simulink model "tqdtqr_rebuild_V3"  (R2021b)
settings: Solver=VariableStepAuto  StartTime=0.0  StopTime=10.0  RelTol=1e-3
undefined symbols (not defined in the file): ATQD_AfterTqMinGain_X_Deg, ATQD_APSCreepBaseTqD_X_kph, ATQD_APSCreepBaseTqD_Y_Deg, ATQD_APSCreepBaseTqR_X_kph, ATQD_APSCreepBaseTqR_Y_Deg, ATQD_APSCreepIterm_X_kph, ATQD_APSCreepIterm_Y_kph, ATQD_APSCreepPterm_X_kph, ATQD_APSCreepPterm_Y_kph, ATQD_APSDecReq_X_kph, ATQD_APSDecReq_Y_mps2, ATQD_APSDecReqCMD_X_kph, ATQD_APSDecReqTs_X_pct, ATQD_APSDecTimeGain_X_Deg, ATQD_APSDecTimeGain_Y_s, ATQD_APSReqLowSpd_X_Deg, ATQD_AutoHoldReleaseBPS_X_Deg, ATQD_AWDLoadTrqnsGain_X_kg, ATQD_AWDLoadTrqnsGain_Y_pct, ATQD_BOSEnBPSPosn_X_kph, ATQD_BOSMap_X_rpm, ATQD_BOSMap_Y_pct, ATQD_CreepBaseTqD_X_kph, ATQD_CreepBaseTqD_Y_Deg, ATQD_CreepBaseTqR_X_kph, ATQD_CreepBaseTqR_Y_Deg, ATQD_CreepBPSDisPosn_X_Deg, ATQD_CreepBPSDisPosnR_X_Deg, ATQD_CreepBPSEnPosn_X_Deg, ATQD_CreepBPSEnPosnR_X_Deg, ATQD_CreepDeltaTq_X_kph, ATQD_CreepIterm_X_kph, ATQD_CreepIterm_Y_kph, ATQD_CreepItermMaxLimit_X_pct, ATQD_CreepPreloadTime_X_kph, ATQD_CreepPreloadTq_X_kph, ATQD_CreepPreloadTq_Y_s, ATQD_CreepProtTq_X_Deg, ATQD_CreepPterm_X_kph, ATQD_CreepPterm_Y_kph, ATQD_CreepRrTqSpRat_X_rpm, ATQD_CreepRrTqSpRat_Y_Nm, ATQD_CreepTargetSpdD_X_pct, ATQD_CreepTargetSpdR_X_pct, ATQD_CreepUpLimitTq_X_rpm, ATQD_DecIneOPDHoldEnDelay_X_Deg, ATQD_DecIneOPDHoldEnDelay_Y_bar, ATQD_ECOTqMapD_X_rpm, ATQD_ECOTqMapD_Y_pct, ATQD_EMTqMapD_X_rpm, ATQD_EMTqMapD_Y_pct, ATQD_EOPDTqMapDCon_X_rpm, ATQD_EOPDTqMapDCon_Y_Deg, ATQD_EstInitVehWeight_X_c, ATQD_FAfterTqCMDGain_X_rpm, ATQD_FAfterTqCMDGain_Y_pct, ATQD_ForceLowSpd_X_Deg, ATQD_ForcePLimitSpd_X_Deg, ATQD_FrLossMAPLowV_X_rpm, ATQD_FrLossMAPLowV_Y_Nm ... (+949)
libraries: simulink x235, hcu_lib x208, tqr x63, tqd x6
(part 4 of 37)

== system tqdtqr_rebuild_V3/Input_Convert/Main function ==
  note: --------------------------------------------------------------------TQR----------------------------------------------------------------
  BSCPIn_outputs : Inport
  BSignalConvert_outputs : Inport  Port=2
  BFunction_outputs : Inport  Port=3
  BMain_outputs : Inport  Port=4
  Add B regen to ramp enable judge : Subsystem
  AvaliableTqLimit function : Subsystem
  Bus Creator : BusCreator  Inputs=72
  DriverWhlTqDem function : Subsystem
  Front/Rear EDU Tq Up/Low Limit : Subsystem
  Front/Rear ramp parameters determine : Subsystem
  Front/Rear wheel torque different function : Subsystem
  Front/Rear wheel torque limitation determine function : Subsystem
  Front/Rear zero point transfer : Subsystem
  Gear detection to inverse motor : Subsystem
  Tq coordination function : Subsystem
  Tq distribution function : Subsystem
  MainFunction_outputs : Outport
  wires:
  [BSCPIn_outputs] -> Tq distribution function/1(BSCPIn_outputs)
  [BSignalConvert_outputs] -> DriverWhlTqDem function/2(BSignalConvert_outputs)
  [BMain_outputs] -> Tq distribution function/2(BMain_outputs)
  [BFunction_outputs] -> Tq distribution function/4(BFunction_outputs)
  [BSignalConvert_outputs] -> Tq distribution function/3(BSignalConvert_outputs)
  [BSCPIn_outputs] -> Tq coordination function/1(BSCPIn_outputs)
  [BSignalConvert_outputs] -> Tq coordination function/2(BSignalConvert_outputs)
  [BFunction_outputs] -> DriverWhlTqDem function/3(BFunction_outputs)
  [BSCPIn_outputs] -> DriverWhlTqDem function/1(BSCPIn_outputs)
  BSCPIn_outputs/1 -> [BSCPIn_outputs]
  BFunction_outputs/1 -> [BFunction_outputs]
  BSignalConvert_outputs/1 -> [BSignalConvert_outputs]
  BMain_outputs/1 -> [BMain_outputs]
  [BMain_outputs] -> Tq coordination function/3(BMain_outputs)
  [BSCPIn_outputs] -> AvaliableTqLimit function/1(BSCPIn_outputs)
  [BSignalConvert_outputs] -> AvaliableTqLimit function/2(BSignalConvert_outputs)
  [BFunction_outputs] -> AvaliableTqLimit function/3(BFunction_outputs)
  [BMain_outputs] -> AvaliableTqLimit function/4(BMain_outputs)
  [BMain_outputs] -> DriverWhlTqDem function/4(BMain_outputs)
  DriverWhlTqDem function/1(VTQD_RollRegenEnable_flg) -> [VTQD_RollRegenEnable_flg]
  DriverWhlTqDem function/2(VTQD_BOSEnable_flg) -> [VTQD_BOSEnable_flg]
  DriverWhlTqDem function/3(VTQD_BOSTq_Nm) -> [VTQD_BOSTq_Nm]
  DriverWhlTqDem function/4(VTQD_IVIRockModeEn_flg) -> [VTQD_IVIRockModeEn_flg]
  DriverWhlTqDem function/5(VTQD_LoSpdBrkCtrl_flg) -> [VTQD_LoSpdBrkCtrl_flg]
  DriverWhlTqDem function/6(VTQD_RockModeTCSReq_flg) -> [VTQD_RockModeTCSReq_flg]
  DriverWhlTqDem function/7(VTQD_RockModePedTq_Nm) -> [VTQD_RockModePedTq_Nm]
  DriverWhlTqDem function/8(VTQD_RockModeTqLim_flg) -> [VTQD_RockModeTqLim_flg]
  DriverWhlTqDem function/9(VTQD_PreLoadPreEn_flg) -> [VTQD_PreLoadPreEn_flg]
  DriverWhlTqDem function/10(VTQD_PreloadTq_Nm) -> [VTQD_PreloadTq_Nm]
  DriverWhlTqDem function/11(VTQD_PreLoadHold_flg) -> [VTQD_PreLoadHold_flg]
  DriverWhlTqDem function/12(VTQD_CreepWhlTqDem_Nm) -> [VTQD_CreepWhlTqDem_Nm]
  DriverWhlTqDem function/13(VTQD_CreepPrLoadEnable_flg) -> [VTQD_CreepPrLoadEnable_flg]
  DriverWhlTqDem function/14(VTQD_CreepProtTqEn_flg) -> [VTQD_CreepProtTqEn_flg]
  DriverWhlTqDem function/15(VTQD_PedalMapWhlTq_Nm) -> [VTQD_PedalMapWhlTq_Nm]
  DriverWhlTqDem function/16(VTQD_EVDriveModeValid_flg) -> [VTQD_EVDriveModeValid_flg]
  DriverWhlTqDem function/17(VTQD_RegenTqLimitEn_flg) -> [VTQD_RegenTqLimitEn_flg]
  DriverWhlTqDem function/18(VTQD_PedAccTqEn_flg) -> [VTQD_PedAccTqEn_flg]
  DriverWhlTqDem function/19(VTQD_SlideRegenLimTq_Nm) -> [VTQD_SlideRegenLimTq_Nm]
  DriverWhlTqDem function/20(VTQD_OPDOn2Off_flg) -> [VTQD_OPDOn2Off_flg]
  DriverWhlTqDem function/21(VTQD_CreepTCSActive_flg) -> [VTQD_CreepTCSActive_flg]
  DriverWhlTqDem function/22(VTQD_FrPreloadTq_Nm) -> [VTQD_FrPreloadTq_Nm]
  DriverWhlTqDem function/23(VTQD_RrPreloadTq_Nm) -> [VTQD_RrPreloadTq_Nm]
  DriverWhlTqDem function/24(VTQD_CreepEnable_flg) -> [VTQD_CreepEnable_flg]
  DriverWhlTqDem function/25(VTQD_CreepBaseTqD_Nm) -> [VTQD_CreepBaseTqD_Nm]
  [VTQD_RollRegenEnable_flg] -> Tq coordination function/4(VTQD_RollRegenEnable_flg)
  [VTQD_CreepPrLoadEnable_flg] -> Tq distribution function/5(VTQD_CreepPrLoadEnable_flg)
  [VTQD_CreepEnable_flg] -> Tq distribution function/6(VTQD_CreepEnable_flg)
  [VTQD_RrPreloadTq_Nm] -> Tq distribution function/7(VTQD_RrPreloadTq_Nm)
  [VTQD_FrPreloadTq_Nm] -> Tq distribution function/8(VTQD_FrPreloadTq_Nm)
  [VTQD_PreLoadHold_flg] -> Tq distribution function/9(VTQD_PreLoadHold_flg)
  Tq coordination function/1(VTQD_TqSourceFr_enum) -> [VTQD_TqSourceFr_enum]
  Tq coordination function/2(VTQD_TqSourceRr_enum) -> [VTQD_TqSourceRr_enum]
  Tq coordination function/3(VTQD_TotalWhlTqCapMot_Nm) -> [VTQD_TotalWhlTqCapMot_Nm]
  Tq coordination function/4(VTQD_TotalWhlTqCapGen_Nm) -> [VTQD_TotalWhlTqCapGen_Nm]
  [VTQD_TqSourceRr_enum] -> DriverWhlTqDem function/6(VTQD_TqSourceRr_enum)
  [VTQD_TqSourceFr_enum] -> DriverWhlTqDem function/5(VTQD_TqSourceFr_enum)
  Tq distribution function/1(VTQD_FrEDUSpRat_rat) -> [VTQD_FrEDUSpRat_rat]
  Tq distribution function/2(VTQD_RrEDUSpRat_rat) -> [VTQD_RrEDUSpRat_rat]
  Tq distribution function/3(VTQD_RockModePedTqFr_Nm) -> [VTQD_RockModePedTqFr_Nm]
  Tq distribution function/4(VTQD_RockModePedTqRr_Nm) -> [VTQD_RockModePedTqRr_Nm]
  Tq distribution function/5(VTQD_TMEnOutpTqSta_enum) -> [VTQD_TMEnOutpTqSta_enum]
  Tq distribution function/6(VTQD_NewDistFrWhlTq_Nm) -> [VTQD_NewDistFrWhlTq_Nm]
  Tq distribution function/7(VTQD_NewDistRrWhlTq_Nm) -> [VTQD_NewDistRrWhlTq_Nm]
  [VTQD_FrEDUSpRat_rat] -> AvaliableTqLimit function/6(VTQD_FrEDUSpRat_rat)
  [VTQD_RrEDUSpRat_rat] -> AvaliableTqLimit function/7(VTQD_RrEDUSpRat_rat)
  AvaliableTqLimit function/1(VTQD_WhlTqCapMotFr_Nm) -> [VTQD_WhlTqCapMotFr_Nm]
  AvaliableTqLimit function/2(VTQD_WhlTqCapMotRr_Nm) -> [VTQD_WhlTqCapMotRr_Nm]
  AvaliableTqLimit function/3(VTQD_WhlTqCapGenFr_Nm) -> [VTQD_WhlTqCapGenFr_Nm]
  AvaliableTqLimit function/4(VTQD_WhlTqCapGenRr_Nm) -> [VTQD_WhlTqCapGenRr_Nm]
  AvaliableTqLimit function/5(VTQD_MotorLossTotal_kw) -> [VTQD_MotorLossTotal_kw]
  AvaliableTqLimit function/6(VTQD_FAfterTqCMDGain_c) -> [VTQD_FAfterTqCMDGain_c]
  AvaliableTqLimit function/7(VTQD_RAfterTqCMDGain_c) -> [VTQD_RAfterTqCMDGain_c]
  [VTQD_MotorLossTotal_kw] -> Tq coordination function/5(VTQD_MotorLossTotal_kw)
  [VTQD_RollRegenEnable_flg] -> Bus Creator/1
  [VTQD_BOSEnable_flg] -> Bus Creator/2
  [VTQD_BOSTq_Nm] -> Bus Creator/3
  [VTQD_IVIRockModeEn_flg] -> Bus Creator/4
  [VTQD_LoSpdBrkCtrl_flg] -> Bus Creator/5
  [VTQD_RockModeTCSReq_flg] -> Bus Creator/6
  [VTQD_RockModePedTq_Nm] -> Bus Creator/7
  [VTQD_RockModeTqLim_flg] -> Bus Creator/8
  [VTQD_PreLoadPreEn_flg] -> Bus Creator/9
  [VTQD_PreloadTq_Nm] -> Bus Creator/10
  [VTQD_PreLoadHold_flg] -> Bus Creator/11
  [VTQD_CreepWhlTqDem_Nm] -> Bus Creator/12
  [VTQD_CreepPrLoadEnable_flg] -> Bus Creator/13
  [VTQD_CreepProtTqEn_flg] -> Bus Creator/14
  [VTQD_PedalMapWhlTq_Nm] -> Bus Creator/15
  [VTQD_EVDriveModeValid_flg] -> Bus Creator/16
  [VTQD_RegenTqLimitEn_flg] -> Bus Creator/17
  [VTQD_PedAccTqEn_flg] -> Bus Creator/18
  [VTQD_SlideRegenLimTq_Nm] -> Bus Creator/19
  [VTQD_OPDOn2Off_flg] -> Bus Creator/20
  [VTQD_CreepTCSActive_flg] -> Bus Creator/21
  [VTQD_FrPreloadTq_Nm] -> Bus Creator/22
  [VTQD_RrPreloadTq_Nm] -> Bus Creator/23
  [VTQD_CreepEnable_flg] -> Bus Creator/24
  [VTQD_CreepBaseTqD_Nm] -> Bus Creator/25
  [VTQD_TqSourceFr_enum] -> Bus Creator/26
  [VTQD_TqSourceRr_enum] -> Bus Creator/27
  [VTQD_TotalWhlTqCapMot_Nm] -> Bus Creator/28
  [VTQD_FrEDUSpRat_rat] -> Bus Creator/31
  [VTQD_RrEDUSpRat_rat] -> Bus Creator/32
  [VTQD_RockModePedTqFr_Nm] -> Bus Creator/33
  [VTQD_RockModePedTqRr_Nm] -> Bus Creator/34
  [VTQD_TMEnOutpTqSta_enum] -> Bus Creator/35
  [VTQD_NewDistFrWhlTq_Nm] -> Bus Creator/36
  [VTQD_NewDistRrWhlTq_Nm] -> Bus Creator/37
  [VTQD_WhlTqCapMotFr_Nm] -> Bus Creator/38
  [VTQD_WhlTqCapMotRr_Nm] -> Bus Creator/39
  [VTQD_WhlTqCapGenFr_Nm] -> Bus Creator/40
  [VTQD_WhlTqCapGenRr_Nm] -> Bus Creator/41
  [VTQD_MotorLossTotal_kw] -> Bus Creator/42
  [VTQD_FAfterTqCMDGain_c] -> Bus Creator/43
  [VTQD_RAfterTqCMDGain_c] -> Bus Creator/44
  Bus Creator/1 -> MainFunction_outputs/1
  [BSCPIn_outputs] -> Front/Rear wheel torque different function/1(BSCPIn_outputs)
  [BSignalConvert_outputs] -> Front/Rear wheel torque different function/2(BSignalConvert_outputs)
  Front/Rear wheel torque different function/1(VTQR_FShaftSpdTqLimCoe_c) -> [VTQR_FShaftSpdTqLimCoe_c]
  Front/Rear wheel torque different function/2(VTQR_FTimerTqLimCoe_c) -> [VTQR_FTimerTqLimCoe_c]
  Front/Rear wheel torque different function/3(VTQR_RShaftSpdTqLimCoe_c) -> [VTQR_RShaftSpdTqLimCoe_c]
  Front/Rear wheel torque different function/4(VTQR_RTimerTqLimCoe_c) -> [VTQR_RTimerTqLimCoe_c]
  [VTQR_FShaftSpdTqLimCoe_c] -> Front/Rear wheel torque limitation determine function/3(VTQR_FShaftSpdTqLimCoe_c)
  [VTQR_FTimerTqLimCoe_c] -> Front/Rear wheel torque limitation determine function/4(VTQR_FTimerTqLimCoe_c)
  [VTQR_RShaftSpdTqLimCoe_c] -> Front/Rear wheel torque limitation determine function/5(VTQR_RShaftSpdTqLimCoe_c)
  [VTQR_RTimerTqLimCoe_c] -> Front/Rear wheel torque limitation determine function/6(VTQR_RTimerTqLimCoe_c)
  [BMain_outputs] -> Front/Rear wheel torque limitation determine function/2(BMain_outputs)
  [BSCPIn_outputs] -> Front/Rear wheel torque limitation determine function/1(BSCPIn_outputs)
  Front/Rear wheel torque limitation determine function/1(VTQR_ActFEDUTrqUpLim_Nm) -> [VTQR_ActFEDUTrqUpLim_Nm]
  Front/Rear wheel torque limitation determine function/2(VTQR_ActFEDUTrqLowLim_Nm) -> [VTQR_ActFEDUTrqLowLim_Nm]
  Front/Rear wheel torque limitation determine function/4(VTQR_ActREDUTrqLowLim_Nm) -> [VTQR_ActREDUTrqLowLim_Nm]
  Front/Rear wheel torque limitation determine function/3(VTQR_ActREDUTrqUpLim_Nm) -> [VTQR_ActREDUTrqUpLim_Nm]
  Front/Rear wheel torque different function/5(VTQR_FShaftSpdTqLimLow_flg) -> [VTQR_FShaftSpdTqLimLow_flg]
  Front/Rear wheel torque different function/6(VTQR_FTimerTqLimLow_flg) -> [VTQR_FTimerTqLimLow_flg]
  Front/Rear wheel torque different function/7(VTQR_RShaftSpdTqLimLow_flg) -> [VTQR_RShaftSpdTqLimLow_flg]
  Front/Rear wheel torque different function/8(VTQR_RTimerTqLimLow_flg) -> [VTQR_RTimerTqLimLow_flg]
  [BSCPIn_outputs] -> Front/Rear zero point transfer/1(BSCPIn_outputs)
  [BMain_outputs] -> Front/Rear zero point transfer/3(BMain_outputs)
  [BSignalConvert_outputs] -> Front/Rear zero point transfer/2(BSignalConvert_outputs)
  [VTQD_CreepPrLoadEnable_flg] -> Front/Rear zero point transfer/4(VTQD_CreepPrLoadEnable_flg)
  [VTQD_PreLoadPreEn_flg] -> Front/Rear zero point transfer/5(VTQD_PreLoadPreEn_flg)
  Front/Rear zero point transfer/1(VTQR_FrTqZeroTransUpBound_Nm) -> [VTQR_FrTqZeroTransUpBound_Nm]
  Front/Rear zero point transfer/2(VTQR_FrTqZeroTransLowBound_Nm) -> [VTQR_FrTqZeroTransLowBound_Nm]
  Front/Rear zero point transfer/3(VTQR_FrTqZeroTrans_enum) -> [VTQR_FrTqZeroTrans_enum]
  Front/Rear zero point transfer/4(VTQR_RrTqZeroTransUpBound_Nm) -> [VTQR_RrTqZeroTransUpBound_Nm]
  Front/Rear zero point transfer/5(VTQR_RrTqZeroTransLowBound_Nm) -> [VTQR_RrTqZeroTransLowBound_Nm]
  Front/Rear zero point transfer/6(VTQR_RrTqZeroTrans_enum) -> [VTQR_RrTqZeroTrans_enum]
  [VTQR_FShaftSpdTqLimLow_flg] -> Bus Creator/45
  [VTQR_FTimerTqLimLow_flg] -> Bus Creator/46
  [VTQR_RShaftSpdTqLimLow_flg] -> Bus Creator/47
  [VTQR_RTimerTqLimLow_flg] -> Bus Creator/48
  [VTQR_ActFEDUTrqUpLim_Nm] -> Bus Creator/49
  [VTQR_ActFEDUTrqLowLim_Nm] -> Bus Creator/50
  [VTQR_ActREDUTrqUpLim_Nm] -> Bus Creator/51
  [VTQR_ActREDUTrqLowLim_Nm] -> Bus Creator/52
  [VTQR_FrTqZeroTransUpBound_Nm] -> Bus Creator/53
  [VTQR_FrTqZeroTransLowBound_Nm] -> Bus Creator/54
  [VTQR_FrTqZeroTrans_enum] -> Bus Creator/55
  [VTQR_RrTqZeroTransUpBound_Nm] -> Bus Creator/56
  [VTQR_RrTqZeroTransLowBound_Nm] -> Bus Creator/57
  [VTQR_RrTqZeroTrans_enum] -> Bus Creator/58
  [BFunction_outputs] -> Gear detection to inverse motor/1(BFunction_outputs)
  [BMain_outputs] -> Gear detection to inverse motor/2(BMain_outputs)
  Gear detection to inverse motor/1(VTQR_FrGearChange_flg) -> [VTQR_FrGearChange_flg]
  Gear detection to inverse motor/2(VTQR_RrGearChange_flg) -> [VTQR_RrGearChange_flg]
  [VTQR_FrGearChange_flg] -> Bus Creator/59
  [VTQR_RrGearChange_flg] -> Bus Creator/60
  [BSignalConvert_outputs] -> Front/Rear ramp parameters determine/2(BSignalConvert_outputs)
  [BSCPIn_outputs] -> Front/Rear ramp parameters determine/1(BSCPIn_outputs)
  [VTQD_RollRegenEnable_flg] -> Front/Rear ramp parameters determine/5(VTQD_RollRegenEnable_flg)
  [VTQD_TqSourceFr_enum] -> Front/Rear ramp parameters determine/6(VTQD_TqSourceFr_enum)
  [BMain_outputs] -> Front/Rear ramp parameters determine/4(BMain_outputs)
  [VTQD_EVDriveModeValid_flg] -> Front/Rear ramp parameters determine/7(VTQD_EVDriveModeValid_flg)
  [VTQD_PreLoadHold_flg] -> Front/Rear ramp parameters determine/8(VTQD_PreLoadHold_flg)
  [VTQD_CreepPrLoadEnable_flg] -> Front/Rear ramp parameters determine/9(VTQD_CreepPrLoadEnable_flg)
  [VTQD_PedAccTqEn_flg] -> Front/Rear ramp parameters determine/10(VTQD_PedAccTqEn_flg)
  [VTQD_PreLoadPreEn_flg] -> Front/Rear ramp parameters determine/11(VTQD_PreLoadPreEn_flg)
  [VTQD_IVIRockModeEn_flg] -> Front/Rear ramp parameters determine/12(VTQD_IVIRockModeEn_flg)
  [VTQR_FrTqZeroTrans_enum] -> Front/Rear ramp parameters determine/13(VTQR_FrTqZeroTrans_enum)
  [VTQD_RegenTqLimitEn_flg] -> Front/Rear ramp parameters determine/14(VTQD_RegenTqLimitEn_flg)
  [BFunction_outputs] -> Front/Rear ramp parameters determine/3(BFunction_outputs)
  [VTQD_TqSourceRr_enum] -> Front/Rear ramp parameters determine/15(VTQD_TqSourceRr_enum)
  [VTQR_RrTqZeroTrans_enum] -> Front/Rear ramp parameters determine/16(VTQR_RrTqZeroTrans_enum)
  Front/Rear ramp parameters determine/1(VTQR_FrFirstOrderInpTs_c) -> [VTQR_FrFirstOrderInpTs_c]
  Front/Rear ramp parameters determine/2(VTQR_FrRateLimitInc_Nm) -> [VTQR_FrRateLimitInc_Nm]
  Front/Rear ramp parameters determine/3(VTQR_FrRateLimitDec_Nm) -> [VTQR_FrRateLimitDec_Nm]
  Front/Rear ramp parameters determine/4(VTQR_RrFirstOrderInpTs_c) -> [VTQR_RrFirstOrderInpTs_c]
  Front/Rear ramp parameters determine/5(VTQR_RrRateLimitInc_Nm) -> [VTQR_RrRateLimitInc_Nm]
  Front/Rear ramp parameters determine/6(VTQR_RrRateLimitDec_Nm) -> [VTQR_RrRateLimitDec_Nm]
  [VTQR_FrFirstOrderInpTs_c] -> Bus Creator/61
  [VTQR_FrRateLimitInc_Nm] -> Bus Creator/62
  [VTQR_FrRateLimitDec_Nm] -> Bus Creator/63
  [VTQR_RrFirstOrderInpTs_c] -> Bus Creator/64
  [VTQR_RrRateLimitInc_Nm] -> Bus Creator/65
  [VTQR_RrRateLimitDec_Nm] -> Bus Creator/66
  [VTQR_FrTqZeroTransLowBound_Nm] -> Tq distribution function/10(VTQR_FrTqZeroTransLowBound_Nm)
  [VTQR_RrTqZeroTransLowBound_Nm] -> Tq distribution function/11(VTQR_RrTqZeroTransLowBound_Nm)
  [VTQR_FShaftSpdTqLimLow_flg] -> DriverWhlTqDem function/7(VTQR_FShaftSpdTqLimLow_flg)
  [VTQR_FTimerTqLimLow_flg] -> DriverWhlTqDem function/8(VTQR_FTimerTqLimLow_flg)
  [VTQR_RShaftSpdTqLimLow_flg] -> DriverWhlTqDem function/9(VTQR_RShaftSpdTqLimLow_flg)
  [VTQR_RTimerTqLimLow_flg] -> DriverWhlTqDem function/10(VTQR_RTimerTqLimLow_flg)
  [BSCPIn_outputs] -> Add B regen to ramp enable judge/1(BSCPIn_outputs)
  [BSignalConvert_outputs] -> Add B regen to ramp enable judge/2(BSignalConvert_outputs)
  [BFunction_outputs] -> Add B regen to ramp enable judge/3(BFunction_outputs)
  Add B regen to ramp enable judge/1(VTQD_FEDUWhlTqBRegen_Nm) -> [VTQD_FEDUWhlTqBRegen_Nm]
  Add B regen to ramp enable judge/2(VTQD_REDUWhlTqBRegen_Nm) -> [VTQD_REDUWhlTqBRegen_Nm]
  [BSCPIn_outputs] -> Front/Rear EDU Tq Up/Low Limit/1(BSCPIn_outputs)
  [BSignalConvert_outputs] -> Front/Rear EDU Tq Up/Low Limit/2(BSignalConvert_outputs)
  [BFunction_outputs] -> Front/Rear EDU Tq Up/Low Limit/3(BFunction_outputs)
  [VTQD_WhlTqCapMotFr_Nm] -> Front/Rear EDU Tq Up/Low Limit/4(VTQD_WhlTqCapMotFr_Nm)
  [VTQD_WhlTqCapMotRr_Nm] -> Front/Rear EDU Tq Up/Low Limit/5(VTQD_WhlTqCapMotRr_Nm)
  [VTQD_WhlTqCapGenFr_Nm] -> Front/Rear EDU Tq Up/Low Limit/6(VTQD_WhlTqCapGenFr_Nm)
  [VTQD_WhlTqCapGenRr_Nm] -> Front/Rear EDU Tq Up/Low Limit/7(VTQD_WhlTqCapGenRr_Nm)
  Front/Rear EDU Tq Up/Low Limit/1(VTQR_ActFEDUTqLowLimit_Nm) -> [VTQR_ActFEDUTqLowLimit_Nm]
  Front/Rear EDU Tq Up/Low Limit/2(VTQR_ActFEDUTqUpLimit_Nm) -> [VTQR_ActFEDUTqUpLimit_Nm]
  Front/Rear EDU Tq Up/Low Limit/3(VTQR_ActREDUTqUpLimit_Nm) -> [VTQR_ActREDUTqUpLimit_Nm]
  Front/Rear EDU Tq Up/Low Limit/4(VTQR_ActREDUTqLowLimit_Nm) -> [VTQR_ActREDUTqLowLimit_Nm]
  [VTQD_FEDUWhlTqBRegen_Nm] -> Bus Creator/67
  [VTQD_REDUWhlTqBRegen_Nm] -> Bus Creator/68
  [VTQR_ActFEDUTqLowLimit_Nm] -> Bus Creator/69
  [VTQR_ActFEDUTqUpLimit_Nm] -> Bus Creator/70
  [VTQR_ActREDUTqUpLimit_Nm] -> Bus Creator/71
  [VTQR_ActREDUTqLowLimit_Nm] -> Bus Creator/72
  Front/Rear zero point transfer/7(VTQD_FrZeroPointIncDec_Nm) -> [VTQD_FrZeroPointIncDec_Nm]
  Front/Rear zero point transfer/8(VTQD_RrZeroPointIncDec_Nm) -> [VTQD_RrZeroPointIncDec_Nm]
  [VTQD_FrZeroPointIncDec_Nm] -> Front/Rear ramp parameters determine/17(VTQD_FrZeroPointIncDec_Nm)
  [VTQD_RrZeroPointIncDec_Nm] -> Front/Rear ramp parameters determine/18(VTQD_RrZeroPointIncDec_Nm)
  [VTQD_IVIRockModeEn_flg] -> AvaliableTqLimit function/5(VTQD_IVIRockModeEn_flg)
  Tq coordination function/5(VTQD_ForceIdleTqReq_Nm) -> [VTQD_ForceIdleTqReq_Nm]
  [VTQD_TotalWhlTqCapGen_Nm] -> Bus Creator/29
  [VTQD_ForceIdleTqReq_Nm] -> Bus Creator/30

== system tqdtqr_rebuild_V3/Input_Convert/Signal function ==
  BSCPIn_outputs : Inport
  BSignalConvert_outputs : Inport  Port=2
  BMain_outputs : Inport  Port=3
  DriverWhlTqDemFunc_outputs : Inport  Port=4
  Bus Creator : BusCreator  Inputs=62
  MCU Damping Disable Judgement : Subsystem
  New Wheel Slide Rate : Subsystem
  OPD Hold : Subsystem
  Regen level define : Subsystem
  SWC1 SWC2 status : Subsystem
  ShiftModule : Subsystem
  Simulation Sound Wave : Subsystem
  VINP_EPBCarWashMode_flg : Subsystem
  VehWeightEst : Subsystem
  Wheel Status Judgment : Subsystem
  combo key : Subsystem
  BFunction_outputs : Outport
  wires:
  BSCPIn_outputs/1 -> [BSCPIn_outputs]
  BSignalConvert_outputs/1 -> [BSignalConvert_outputs]
  BMain_outputs/1 -> [BMain_outputs]
  [BSCPIn_outputs] -> Regen level define/1(BSCPIn_outputs)
  [BSignalConvert_outputs] -> Regen level define/2(BSignalConvert_outputs)
  [BSCPIn_outputs] -> New Wheel Slide Rate/1(BSCPIn_outputs)
  [BMain_outputs] -> New Wheel Slide Rate/2(BMain_outputs)
  New Wheel Slide Rate/1(VTQD_MaxWhlSlideRate_pct) -> [VTQD_MaxWhlSlideRate_pct]
  [VTQD_LFSlideRate_pct] -> Regen level define/3(VTQD_LFSlideRate_pct)
  [BSCPIn_outputs] -> Simulation Sound Wave/1(BSCPIn_outputs)
  [BSCPIn_outputs] -> Wheel Status Judgment/1(BSCPIn_outputs)
  [BMain_outputs] -> Wheel Status Judgment/3(BMain_outputs)
  [BSignalConvert_outputs] -> Wheel Status Judgment/2(BSignalConvert_outputs)
  [BSCPIn_outputs] -> VehWeightEst/1(BSCPIn_outputs)
  [BMain_outputs] -> VehWeightEst/3(BMain_outputs)
  [BSignalConvert_outputs] -> VehWeightEst/2(BSignalConvert_outputs)
  [BSCPIn_outputs] -> ShiftModule/1(BSCPIn_outputs)
  [BSignalConvert_outputs] -> ShiftModule/2(BSignalConvert_outputs)
  [BMain_outputs] -> ShiftModule/7(BMain_outputs)
  SWC1 SWC2 status/1(VTQD_SWCResUpSta_flg) -> [VTQD_SWCResUpSta_flg]
  [SWC_RegenUp] -> ShiftModule/4(SWC_RegenUp)
  [VTQD_GearActualPosn_enum] -> VehWeightEst/4(VTQD_GearActualPosn_enum)
  [VTQD_FDCVCURegenMode_enum] -> VehWeightEst/5(VTQD_FDCVCURegenMode_enum)
  VehWeightEst/1(VTQD_EstVehWeightResult_kg) -> [VTQD_EstVehWeightResult_kg]
  [VTQD_GearActualPosn_enum] -> Regen level define/7(VTQD_GearActualPosn_enum)
  [VTQD_GearActualPosn_enum] -> Simulation Sound Wave/2(VTQD_GearActualPosn_enum)
  Simulation Sound Wave/1(VTQD_SimSouWaveReq_pct) -> [SimulationSoundWave_outputs]
  [VTQD_GearActualPosn_enum] -> Wheel Status Judgment/4(VTQD_GearActualPosn_enum)
  Wheel Status Judgment/1(VTQD_ActWhlSkipSta_enum) -> [VTQD_ActWhlSkipSta_enum]
  ShiftModule/6(VTQD_DriveProtEn_flg) -> [VTQD_DriveProtEn_flg]
  ShiftModule/7(VTQD_ForceP_flg) -> [VTQD_ForceP_flg]
  ShiftModule/5(VTQD_DriveProtRemove_flg) -> [VTQD_DriveProtRemove_flg]
  ShiftModule/4(VTQD_PBWUnlockTO_flg) -> [VTQD_PBWUnlockTO_flg]
  ShiftModule/3(VTQD_PBWLockTO_flg) -> [VTQD_PBWLockTO_flg]
  ShiftModule/2(VTQD_ParkRequest_flg) -> [VTQD_ParkRequest_flg]
  SWC1 SWC2 status/2(VTQD_SWCSetdownSta_flg) -> [VTQD_SWCSetdownSta_flg]
  SWC1 SWC2 status/3(VTQD_SWCCancelSta_flg) -> [VTQD_SWCCancelSta_flg]
  Regen level define/1(SWC_RegenUp) -> [SWC_RegenUp]
  Regen level define/2(SWC_RegenDown) -> [SWC_RegenDown]
  Regen level define/3(VTQD_FDCVCURegenMode_enum) -> [VTQD_FDCVCURegenMode_enum]
  Regen level define/4(VTQD_SaveRegenMode_enum) -> [VTQD_SaveRegenMode_enum]
  Regen level define/5(VTQD_TrailerDisOPDSta_flg) -> [VTQD_TrailerDisOPDSta_flg]
  SWC1 SWC2 status/4(VTQD_SpdCtrlMode_enum) -> [VTQD_SpdCtrlMode_enum]
  SWC1 SWC2 status/5(VTQD_SpdCtrlSta_flg) -> [VTQD_SpdCtrlSta_flg]
  SWC1 SWC2 status/6(VTQD_SetSpd_kph) -> [VTQD_SetSpd_kph]
  SWC1 SWC2 status/7(VTQD_SWC2ResUpSta_flg) -> [VTQD_SWC2ResUpSta_flg]
  SWC1 SWC2 status/8(VTQD_SWC2SetdownSta_flg) -> [VTQD_SWC2SetdownSta_flg]
  SWC1 SWC2 status/9(VTQD_SWC2CancelSta_flg) -> [VTQD_SWC2CancelSta_flg]
  SWC1 SWC2 status/10(VTQD_SWC2LADASSta_flg) -> [VTQD_SWC2LADASSta_flg]
  SWC1 SWC2 status/11(VTQD_SpdLim4SetSpd_raw32) -> [VTQD_SpdLim4SetSpd_raw32]
  [SWC_RegenDown] -> ShiftModule/5(SWC_RegenDown)
  New Wheel Slide Rate/2(VTQD_MinWhlSlideRate_pct) -> [VTQD_MinWhlSlideRate_pct]
  New Wheel Slide Rate/3(VTQD_LeftSlideRate_pct) -> [VTQD_LeftSlideRate_pct]
  New Wheel Slide Rate/4(VTQD_RightSlideRate_pct) -> [VTQD_RightSlideRate_pct]
  New Wheel Slide Rate/5(VTQD_FrontSlideRate_pct) -> [VTQD_FrontSlideRate_pct]
  New Wheel Slide Rate/6(VTQD_RearSlideRate_pct) -> [VTQD_RearSlideRate_pct]
  New Wheel Slide Rate/7(VTQD_LFSlideRate_pct) -> [VTQD_LFSlideRate_pct]
  New Wheel Slide Rate/8(VTQD_LRSlideRate_pct) -> [VTQD_LRSlideRate_pct]
  New Wheel Slide Rate/9(VTQD_RFSlideRate_pct) -> [VTQD_RFSlideRate_pct]
  New Wheel Slide Rate/10(VTQD_RRSlideRate_pct) -> [VTQD_RRSlideRate_pct]
  [VTQD_RRSlideRate_pct] -> Regen level define/6(VTQD_RRSlideRate_pct)
  [VTQD_LRSlideRate_pct] -> Regen level define/5(VTQD_LRSlideRate_pct)
  [VTQD_RFSlideRate_pct] -> Regen level define/4(VTQD_RFSlideRate_pct)
  Simulation Sound Wave/2(VTQD_SimSoundCmd_pct) -> [VTQD_SimSoundCmd_pct]
  Wheel Status Judgment/2(VTQD_SkipDirect_enum) -> [VTQD_SkipDirect_enum]
  [VTQD_EstVehWeightResult_kg] -> Bus Creator/1
  [VTQD_SWCResUpSta_flg] -> Bus Creator/2
  [VTQD_SWCSetdownSta_flg] -> Bus Creator/3
  [VTQD_SWCCancelSta_flg] -> Bus Creator/4
  [SWC_RegenUp] -> Bus Creator/5
  [SWC_RegenDown] -> Bus Creator/6
  [VTQD_FDCVCURegenMode_enum] -> Bus Creator/7
  [VTQD_SaveRegenMode_enum] -> Bus Creator/8
  [VTQD_TrailerDisOPDSta_flg] -> Bus Creator/9
  [VTQD_SpdCtrlMode_enum] -> Bus Creator/10
  [VTQD_SpdCtrlSta_flg] -> Bus Creator/11
  [VTQD_SetSpd_kph] -> Bus Creator/12
  [VTQD_SWC2ResUpSta_flg] -> Bus Creator/13
  [VTQD_SWC2SetdownSta_flg] -> Bus Creator/14
  [VTQD_SWC2CancelSta_flg] -> Bus Creator/15
  [VTQD_SWC2LADASSta_flg] -> Bus Creator/16
  [VTQD_SpdLim4SetSpd_raw32] -> Bus Creator/17
  [VTQD_ComboKeyPreEn_flg] -> Bus Creator/18
  [VTQD_ComboKeyEn_flg] -> Bus Creator/19
  [VTQD_SysMode_enum] -> Bus Creator/20
  [VTQD_MaxWhlSlideRate_pct] -> Bus Creator/22
  [VTQD_MinWhlSlideRate_pct] -> Bus Creator/23
  [VTQD_LeftSlideRate_pct] -> Bus Creator/24
  [VTQD_RightSlideRate_pct] -> Bus Creator/25
  [VTQD_FrontSlideRate_pct] -> Bus Creator/26
  [VTQD_RearSlideRate_pct] -> Bus Creator/27
  [VTQD_LFSlideRate_pct] -> Bus Creator/28
  [VTQD_LRSlideRate_pct] -> Bus Creator/29
  [VTQD_RFSlideRate_pct] -> Bus Creator/30
  [VTQD_RRSlideRate_pct] -> Bus Creator/31
  [SimulationSoundWave_outputs] -> Bus Creator/32
  [VTQD_SimSoundCmd_pct] -> Bus Creator/33
  [VTQD_ActWhlSkipSta_enum] -> Bus Creator/34
  [VTQD_SkipDirect_enum] -> Bus Creator/35
  [VTQD_GearActualPosn_enum] -> Bus Creator/36
  [VTQD_ParkRequest_flg] -> Bus Creator/37
  [VTQD_PBWLockTO_flg] -> Bus Creator/38
  [VTQD_PBWUnlockTO_flg] -> Bus Creator/39
  [VTQD_DriveProtRemove_flg] -> Bus Creator/40
  [VTQD_DriveProtEn_flg] -> Bus Creator/41
  [VTQD_ForceP_flg] -> Bus Creator/42
  Bus Creator/1 -> BFunction_outputs/1
  ShiftModule/1(VTQD_GearActualPosn_enum) -> [VTQD_GearActualPosn_enum]
  [BSCPIn_outputs] -> MCU Damping Disable Judgement/1(BSCPIn_outputs)
  [BSignalConvert_outputs] -> MCU Damping Disable Judgement/2(BSignalConvert_outputs)
  MCU Damping Disable Judgement/1(VTQD_FrActvDmpDisabReq_flg) -> [VTQD_FrActvDmpDisabReq_flg]
  MCU Damping Disable Judgement/2(VTQD_RrActvDmpDisabReq_flg) -> [VTQD_RrActvDmpDisabReq_flg]
  [BSCPIn_outputs] -> VINP_EPBCarWashMode_flg/1(BSCPIn_outputs)
  VINP_EPBCarWashMode_flg/1(VTQD_EPBCarWashMode_flg) -> [VTQD_EPBCarWashMode_flg]
  [VTQD_FrActvDmpDisabReq_flg] -> Bus Creator/45
  [VTQD_RrActvDmpDisabReq_flg] -> Bus Creator/46
  [VTQD_EPBCarWashMode_flg] -> ShiftModule/3(VTQD_EPBCarWashMode_flg)
  [VTQD_EPBCarWashMode_flg] -> Bus Creator/47
  [BSCPIn_outputs] -> SWC1 SWC2 status/1(BSCPIn_outputs)
  [BSignalConvert_outputs] -> SWC1 SWC2 status/2(BSignalConvert_outputs)
  [VTQD_GearActualPosn_enum] -> SWC1 SWC2 status/3(VTQD_GearActualPosn_enum)
  SWC1 SWC2 status/12(VTQD_SWC2ScrollUpSta_flg) -> [VTQD_SWC2ScrollUpSta_flg]
  [VTQD_SWC2ScrollUpSta_flg] -> Bus Creator/21
  [BSCPIn_outputs] -> combo key/1(BSCPIn_outputs)
  [BSignalConvert_outputs] -> combo key/2(BSignalConvert_outputs)
  combo key/1(VTQD_ComboKeyPreEn_flg) -> [VTQD_ComboKeyPreEn_flg]
  combo key/2(VTQD_ComboKeyEn_flg) -> [VTQD_ComboKeyEn_flg]
  combo key/3(VTQD_SysMode_enum) -> [VTQD_SysMode_enum]
  SWC1 SWC2 status/14(VTQD_SWC2SetSpd_kph) -> [VTQD_SWC2SetSpd_kph]
  SWC1 SWC2 status/13(VTQD_SWC1SetSpd_kph) -> [VTQD_SWC1SetSpd_kph]
  [VTQD_SWC1SetSpd_kph] -> Bus Creator/48
  [VTQD_SWC2SetSpd_kph] -> Bus Creator/49
  DriverWhlTqDemFunc_outputs/1 -> [DriverWhlTqDemFunc_outputs]
  [DriverWhlTqDemFunc_outputs] -> ShiftModule/6(DriverWhlTqDemFunc_outputs)
  [BSignalConvert_outputs] -> OPD Hold/2(BSignalConvert_outputs)
  [DriverWhlTqDemFunc_outputs] -> OPD Hold/3(DriverWhlTqDemFunc_outputs)
  [BSCPIn_outputs] -> OPD Hold/1(BSCPIn_outputs)
  [VTQD_GearActualPosn_enum] -> OPD Hold/5(VTQD_GearActualPosn_enum)
  [VTQD_ActWhlSkipSta_enum] -> OPD Hold/6(VTQD_ActWhlSkipSta_enum)
  [VTQD_SkipDirect_enum] -> OPD Hold/7(VTQD_SkipDirect_enum)
  [VTQD_ParkRequest_flg] -> OPD Hold/8(VTQD_ParkRequest_flg)
  OPD Hold/1(VTQD_APSStaSys_enum) -> [VTQD_APSStaSys_enum]
  OPD Hold/2(VTQD_APSReq_enum) -> [VTQD_APSReq_enum]
  OPD Hold/3(VTQD_APSDecReqA_flg) -> [VTQD_APSDecReqA_flg]
  OPD Hold/4(VTQD_APSDecReq_mps2) -> [VTQD_APSDecReq_mps2]
  OPD Hold/5(VTQD_ActParkRequest_flg) -> [VTQD_ActParkRequest_flg]
  OPD Hold/6(VTQD_APSReqTimer_s) -> [VTQD_APSReqTimer_s]
  OPD Hold/7(VTQD_OPDHoldEnRel_flg) -> [VTQD_OPDHoldEnRel_flg]
  OPD Hold/8(VTQD_OPDHoldAllowPark_flg) -> [VTQD_OPDHoldAllowPark_flg]
  OPD Hold/9(VTQD_OPDHoldLamp_flg) -> [VTQD_OPDHoldLamp_flg]
  OPD Hold/10(VTQD_OPDHoldActRelTq_Nm) -> [VTQD_OPDHoldActRelTq_Nm]
  OPD Hold/11(VTQD_OPDHoldDelayForP_flg) -> [VTQD_OPDHoldDelayForP_flg]
  [VTQD_APSStaSys_enum] -> Bus Creator/50
  [VTQD_APSReq_enum] -> Bus Creator/51
  [VTQD_APSDecReqA_flg] -> Bus Creator/52
  [VTQD_APSDecReq_mps2] -> Bus Creator/53
  [VTQD_ActParkRequest_flg] -> Bus Creator/54
  [VTQD_APSReqTimer_s] -> Bus Creator/55
  [VTQD_OPDHoldEnRel_flg] -> Bus Creator/56
  [VTQD_OPDHoldAllowPark_flg] -> Bus Creator/57
  [VTQD_OPDHoldActRelTq_Nm] -> Bus Creator/59
  [VTQD_OPDHoldLamp_flg] -> Bus Creator/58
  [VTQD_OPDHoldDelayForP_flg] -> Bus Creator/60
  [BMain_outputs] -> OPD Hold/4(BMain_outputs)
  [VTQD_OPDHoldAllowPark_flg] -> ShiftModule/8(VTQD_OPDHoldAllowPark_flg)
  ShiftModule/9(VTQD_ForcePLimitSpd_kph) -> [VTQD_ForcePLimitSpd_kph]
  ShiftModule/8(VTQD_DOALatchReq_flg) -> [VTQD_DOALatchReq_flg]
  [VTQD_DOALatchReq_flg] -> Bus Creator/43
  [VTQD_ForcePLimitSpd_kph] -> Bus Creator/44
  [VTQD_ForceP_flg] -> OPD Hold/9(VTQD_ForceP_flg)
  [VTQD_EPBCarWashMode_flg] -> OPD Hold/10(VTQD_EPBCarWashMode_flg)
  OPD Hold/12(VTQD_OPDHoldAlarm_flg) -> [VTQD_OPDHoldAlarm_flg]
  OPD Hold/13(VTQD_OPDHoldForceEn_flg) -> [VTQD_OPDHoldForceEn_flg]
  [VTQD_OPDHoldAlarm_flg] -> Bus Creator/61
  [VTQD_OPDHoldForceEn_flg] -> Bus Creator/62
  [VTQD_DOALatchReq_flg] -> Regen level define/8(VTQD_DOALatchReq_flg)

== system tqdtqr_rebuild_V3/Main/Avaliable Tq Limit ==
  BSCPIn_outputs : Inport
  BInpConvert_outputs : Inport  Port=2
  VTQD_CoordWhlTqDemFr_Nm : Inport  Port=3
  VTQD_CoordWhlTqDemRr_Nm : Inport  Port=4
  AND{,1..3} (4 alike) : Logic  AllPortsSameDT=off  OutDataTypeStr=boolean
  Bus Selector : BusSelector  OutputSignals=VTQD_WhlTqCapMotFr_Nm,VTQD_WhlTqCapGenFr_Nm,VTQD_PreLoadPreEn_flg,VTQD_DriveProtRemove_flg,VTQD_GearActualPosn_enum,VTQD_FAfterTqCMDGain_c,VTQD_IVIRockModeEn_flg,VTQD_WhlTqCapMotRr_Nm,VTQD_WhlTqCapGenRr_Nm,VTQD_RAfterTqCMDGain_c
  Bus Selector1 : BusSelector  OutputSignals=VINP_FrntAxlTrqReqDrv_Nm,VINP_FrPTCSActive_flg,VVMC_CAASActive_flg,VINP_IVISnowModeCmd_flg,VINP_RearAxlTrqReqDrv_Nm,VINP_RrPTCSActive_flg
  Constant16 : Constant  Value=ZERO_FLOAT
  Constant19 : Constant  Value=ZERO_FLOAT
  Constant21 : Constant  Value=ENUM_GEARACTUALPOSN_N
  Constant22 : Constant  Value=ENUM_GEARACTUALPOSN_P
  Constant23 : Constant  Value=ENUM_GEARACTUALPOSN_N
  Constant24 : Constant  Value=ENUM_GEARACTUALPOSN_P
  Constant25 : Constant  Value=ONE_FLOAT
  Constant26 : Constant  Value=ONE_FLOAT
  Equal{6..9} (4 alike) : RelationalOperator  Operator===  OutDataTypeStr=boolean  RndMeth=Simplest
  Min : MinMax  Inputs=2
  Min1 : MinMax  Inputs=2
  NOT{,1..3} (4 alike) : Logic  Operator=NOT  AllPortsSameDT=off  OutDataTypeStr=boolean
  OR : Logic  Operator=OR  Inputs=4  AllPortsSameDT=off  OutDataTypeStr=boolean
  OR1 : Logic  Operator=OR  Inputs=4  AllPortsSameDT=off  OutDataTypeStr=boolean
  Product : Product
  Product1 : Product
  Saturation Dynamic : simulink/Discontinuities/Saturation Dynamic  OutMin=[]  OutMax=[]  OutDataTypeStr=Inherit: Same as second input  OutDataType=fixdt(1, 16)  OutScaling=2^-10  DoSatur=off
  Saturation Dynamic1 : simulink/Discontinuities/Saturation Dynamic  OutMin=[]  OutMax=[]  OutDataTypeStr=Inherit: Same as second input  OutDataType=fixdt(1, 16)  OutScaling=2^-10  DoSatur=off
  Switch{5..10} (6 alike) : Switch  Criteria=u2 > Threshold
  VTQD_AfterAvailableTqDemFr_Nm : Outport
  VTQD_AfterAvailableTqDemRr_Nm : Outport  Port=2
  wires:
  BInpConvert_outputs/1 -> Bus Selector/1
  [VTQD_IVIRockModeEn_flg] -> NOT2/1
  [VTQD_GearActualPosn_enum] -> Equal6/1
  Equal7/1 -> OR/4
  Constant21/1 -> Equal6/2
  Switch9/1 -> Product/2
  Product/1 -> [VTQD_AfterAvailableTqDemFr_Nm]  "VTQD_AfterAvailableTqDemFr_Nm"
  Constant25/1 -> Switch9/3
  NOT2/1 -> AND2/1
  AND2/1 -> Switch9/2
  Min/1 -> Switch7/1
  [VINP_FrntAxlTrqReqDrv_Nm] -> Min/1
  Equal6/1 -> OR/3
  Constant22/1 -> Equal7/2
  [VTQD_WhlTqCapMotFr_Nm] -> Min/2
  AND/1 -> OR/1
  [VTQD_WhlTqCapMotFr_Nm] -> Switch7/3
  Switch7/1 -> Saturation Dynamic/1  "VTQD_FrAvailableTqUpLimt_Nm"
  [VTQD_CoordWhlTqDemFr_Nm] -> Saturation Dynamic/2
  [VTQD_DriveProtRemove_flg] -> OR/2
  Saturation Dynamic/1 -> Switch5/3
  Constant16/1 -> Switch5/1
  OR/1 -> Switch5/2
  [VVMC_CAASActive_flg] -> AND/2
  [VTQD_PreLoadPreEn_flg] -> NOT/1
  [VTQD_WhlTqCapGenFr_Nm] -> Saturation Dynamic/3
  [VINP_FrPTCSActive_flg] -> Switch7/2
  Switch5/1 -> Product/1
  [VTQD_FAfterTqCMDGain_c] -> Switch9/1
  [VTQD_GearActualPosn_enum] -> Equal7/1
  [VINP_IVISnowModeCmd_flg] -> AND2/2
  NOT/1 -> AND/1
  AND1/1 -> OR1/1
  Constant23/1 -> Equal8/2
  Constant24/1 -> Equal9/2
  Equal8/1 -> OR1/3
  AND3/1 -> Switch10/2
  [VTQD_IVIRockModeEn_flg] -> NOT3/1
  Min1/1 -> Switch8/1
  Saturation Dynamic1/1 -> Switch6/3
  [VTQD_PreLoadPreEn_flg] -> NOT1/1
  Equal9/1 -> OR1/4
  [VTQD_DriveProtRemove_flg] -> OR1/2
  [VINP_RearAxlTrqReqDrv_Nm] -> Min1/1
  [VVMC_CAASActive_flg] -> AND1/2
  [VTQD_WhlTqCapGenRr_Nm] -> Saturation Dynamic1/3
  Switch8/1 -> Saturation Dynamic1/1  "VTQD_RrAvailableTqUpLimt_Nm"
  [VTQD_WhlTqCapMotRr_Nm] -> Switch8/3
  [VTQD_WhlTqCapMotRr_Nm] -> Min1/2
  [VTQD_CoordWhlTqDemRr_Nm] -> Saturation Dynamic1/2
  Switch10/1 -> Product1/2
  [VINP_IVISnowModeCmd_flg] -> AND3/2
  [VTQD_GearActualPosn_enum] -> Equal9/1
  [VTQD_RAfterTqCMDGain_c] -> Switch10/1
  Constant19/1 -> Switch6/1
  [VTQD_GearActualPosn_enum] -> Equal8/1
  NOT3/1 -> AND3/1
  NOT1/1 -> AND1/1
  Product1/1 -> [VTQD_AfterAvailableTqDemRr_Nm]  "VTQD_AfterAvailableTqDemRr_Nm"
  OR1/1 -> Switch6/2
  Switch6/1 -> Product1/1
  [VINP_RrPTCSActive_flg] -> Switch8/2
  Constant26/1 -> Switch10/3
  BSCPIn_outputs/1 -> Bus Selector1/1
  Bus Selector1/1 -> [VINP_FrntAxlTrqReqDrv_Nm]  "<VINP_FrntAxlTrqReqDrv_Nm>"
  Bus Selector/1 -> [VTQD_WhlTqCapMotFr_Nm]  "<VTQD_WhlTqCapMotFr_Nm>"
  Bus Selector1/2 -> [VINP_FrPTCSActive_flg]  "<VINP_FrPTCSActive_flg>"
  VTQD_CoordWhlTqDemFr_Nm/1 -> [VTQD_CoordWhlTqDemFr_Nm]
  Bus Selector/2 -> [VTQD_WhlTqCapGenFr_Nm]  "<VTQD_WhlTqCapGenFr_Nm>"
  Bus Selector/3 -> [VTQD_PreLoadPreEn_flg]  "<VTQD_PreLoadPreEn_flg>"
  Bus Selector1/3 -> [VVMC_CAASActive_flg]  "<VVMC_CAASActive_flg>"
  Bus Selector/4 -> [VTQD_DriveProtRemove_flg]  "<VTQD_DriveProtRemove_flg>"
  Bus Selector/5 -> [VTQD_GearActualPosn_enum]  "<VTQD_GearActualPosn_enum>"
  Bus Selector1/4 -> [VINP_IVISnowModeCmd_flg]  "<VINP_IVISnowModeCmd_flg>"
  Bus Selector/6 -> [VTQD_FAfterTqCMDGain_c]  "<VTQD_FAfterTqCMDGain_c>"
  Bus Selector/7 -> [VTQD_IVIRockModeEn_flg]  "<VTQD_IVIRockModeEn_flg>"
  VTQD_CoordWhlTqDemRr_Nm/1 -> [VTQD_CoordWhlTqDemRr_Nm]
  Bus Selector1/5 -> [VINP_RearAxlTrqReqDrv_Nm]  "<VINP_RearAxlTrqReqDrv_Nm>"
  Bus Selector1/6 -> [VINP_RrPTCSActive_flg]  "<VINP_RrPTCSActive_flg>"
  Bus Selector/8 -> [VTQD_WhlTqCapMotRr_Nm]  "<VTQD_WhlTqCapMotRr_Nm>"
  Bus Selector/9 -> [VTQD_WhlTqCapGenRr_Nm]  "<VTQD_WhlTqCapGenRr_Nm>"
  Bus Selector/10 -> [VTQD_RAfterTqCMDGain_c]  "<VTQD_RAfterTqCMDGain_c>"
  [VTQD_AfterAvailableTqDemFr_Nm] -> VTQD_AfterAvailableTqDemFr_Nm/1
  [VTQD_AfterAvailableTqDemRr_Nm] -> VTQD_AfterAvailableTqDemRr_Nm/1

== system tqdtqr_rebuild_V3/Main/DriverWhlTqDem ==
  BSCPIn_outputs : Inport
  BInpConvert_outputs : Inport  Port=2
  AND10 : Logic  AllPortsSameDT=off  OutDataTypeStr=boolean
  AND14 : Logic  AllPortsSameDT=off  OutDataTypeStr=boolean
  Bus Selector : BusSelector  OutputSignals=VVMC_APSActive_flg
  Bus Selector1 : BusSelector  OutputSignals=VTQD_PreloadTq_Nm,VTQD_PreLoadHold_flg,VTQD_GearActualPosn_enum,VTQD_CreepWhlTqDem_Nm,VTQD_CreepPrLoadEnable_flg,VTQD_CreepProtTqEn_flg,VTQD_LowIdleAccPedal_flg,VTQD_PedalMapWhlTq_Nm,VTQD_PreLoadPreEn_flg,VTQD_RockModePedTq_Nm,VTQD_RockModeTqLim_flg,VTQD_LoSpdBrkCtrl_flg,VTQD_BOSTq_Nm,VTQD_BOSEnable_flg
  Constant10 : Constant  Value=ZERO_FLOAT
  Constant2 : Constant  Value=ZERO_FLOAT
  Constant39 : Constant  Value=KTQD_RocModeTqCtrlSW_flg
  Constant44 : Constant  Value=KTQD_NewPrelaodSW_flg
  Constant8 : Constant  Value=ENUM_GEARACTUALPOSN_P
  Equal9 : RelationalOperator  Operator=~=  OutDataTypeStr=boolean  RndMeth=Simplest
  Logical Operator : Logic  Inputs=3  AllPortsSameDT=off  OutDataTypeStr=boolean
  NOT11 : Logic  Operator=NOT  AllPortsSameDT=off  OutDataTypeStr=boolean
  NOT12 : Logic  Operator=NOT  AllPortsSameDT=off  OutDataTypeStr=boolean
  OR : Logic  Operator=OR  Inputs=3  AllPortsSameDT=off  OutDataTypeStr=boolean
  Switch : Switch  Criteria=u2 ~= 0
  Switch1 : Switch  Criteria=u2 ~= 0
      settings: AttributesFormatString=<%<Criteria>>
  Switch2 : Switch  Criteria=u2 ~= 0  OutDataTypeStr=boolean
      settings: AttributesFormatString=%<Criteria>
  Switch3 : Switch  Criteria=u2 ~= 0
      settings: AttributesFormatString=%<Criteria>
  Switch4 : Switch  Criteria=u2 ~= 0  OutDataTypeStr=boolean
      settings: AttributesFormatString=%<Criteria>
  Switch7 : Switch  Criteria=u2 > Threshold
  VTQD_DriverWhlTqDem_Nm : Outport
  wires:
  BSCPIn_outputs/1 -> Bus Selector/1
  BInpConvert_outputs/1 -> Bus Selector1/1
  Switch1/1 -> [VTQD_DriverWhlTqDem_Nm]  "VTQD_DriverWhlTqDem_Nm"
  Switch4/1 -> Switch7/3
  NOT11/1 -> AND14/2
  Switch3/1 -> Switch4/1
  [VTQD_PreloadTq_Nm] -> Switch3/1
  [VTQD_EscapModeTqLim_flg] -> AND14/1
  [VTQD_EscapeModePedTq_Nm] -> Switch7/1
  AND10/1 -> OR/3
  [VTQD_GearActualPosn_enum] -> Equal9/1
  NOT12/1 -> Logical Operator/3
  Constant2/1 -> Switch3/3
  Constant44/1 -> NOT12/1
  [VTQD_BOSEnable_flg] -> Switch1/2
  [VTQD_CreepPrLoadEnable_flg] -> OR/1
  [VTQD_PreLoadHold_flg] -> Logical Operator/1
  Switch/1 -> Switch1/3
  [VTQD_CreepWhlTqDem_Nm] -> Switch2/1
  Constant10/1 -> Switch/1
  [VVMC_APSActive_flg] -> OR/2
  [VTQD_PedalMapWhlTq_Nm] -> Switch2/3
  [VTQD_BOSTq_Nm] -> Switch1/1
  [VTQD_LowIdleAccPedal_flg] -> AND10/2
  OR/1 -> Switch2/2
  Constant39/1 -> NOT11/1
  [VTQD_CreepProtTqEn_flg] -> AND10/1
  AND14/1 -> Switch7/2
  Logical Operator/1 -> Switch3/2
  [VTQD_LoSpdBrkCtrl_flg] -> Switch/2
  Equal9/1 -> Logical Operator/2
  Switch7/1 -> Switch/3
  [VTQD_PreLoadPreEn_flg] -> Switch4/2
  Switch2/1 -> Switch4/3
  Constant8/1 -> Equal9/2
  [VTQD_DriverWhlTqDem_Nm] -> VTQD_DriverWhlTqDem_Nm/1  "VTQD_DriverWhlTqDem_Nm"
  Bus Selector/1 -> [VVMC_APSActive_flg]  "<VVMC_APSActive_flg>"
  Bus Selector1/1 -> [VTQD_PreloadTq_Nm]  "<VTQD_PreloadTq_Nm>"
  Bus Selector1/2 -> [VTQD_PreLoadHold_flg]  "<VTQD_PreLoadHold_flg>"
  Bus Selector1/3 -> [VTQD_GearActualPosn_enum]  "<VTQD_GearActualPosn_enum>"
  Bus Selector1/4 -> [VTQD_CreepWhlTqDem_Nm]  "<VTQD_CreepWhlTqDem_Nm>"
  Bus Selector1/5 -> [VTQD_CreepPrLoadEnable_flg]  "<VTQD_CreepPrLoadEnable_flg>"
  Bus Selector1/6 -> [VTQD_CreepProtTqEn_flg]  "<VTQD_CreepProtTqEn_flg>"
  Bus Selector1/7 -> [VTQD_LowIdleAccPedal_flg]  "<VTQD_LowIdleAccPedal_flg>"
  Bus Selector1/8 -> [VTQD_PedalMapWhlTq_Nm]  "<VTQD_PedalMapWhlTq_Nm>"
  Bus Selector1/9 -> [VTQD_PreLoadPreEn_flg]  "<VTQD_PreLoadPreEn_flg>"
  Bus Selector1/10 -> [VTQD_EscapeModePedTq_Nm]  "<VTQD_RockModePedTq_Nm>"
  Bus Selector1/11 -> [VTQD_EscapModeTqLim_flg]  "<VTQD_RockModeTqLim_flg>"
  Bus Selector1/12 -> [VTQD_LoSpdBrkCtrl_flg]  "<VTQD_LoSpdBrkCtrl_flg>"
  Bus Selector1/13 -> [VTQD_BOSTq_Nm]  "<VTQD_BOSTq_Nm>"
  Bus Selector1/14 -> [VTQD_BOSEnable_flg]  "<VTQD_BOSEnable_flg>"

== system tqdtqr_rebuild_V3/Main/Front//Rear final torque ==
  note: Rear
  note: Front
  BSCPIn_outputs : Inport
  BInpConvert_outputs : Inport  Port=2
  VTQR_FrFirstOrderInpTq_Nm : Inport  Port=3
  VTQR_RrFirstOrderInpTq_Nm : Inport  Port=4
  Bus Selector : BusSelector  OutputSignals=VTQR_FrFirstOrderInpTs_c,VTQR_FrRateLimitInc_Nm,VTQR_FrRateLimitDec_Nm,VTQR_ActFEDUTrqUpLim_Nm,VTQR_ActFEDUTrqLowLim_Nm,VTQR_RrFirstOrderInpTs_c,VTQR_RrRateLimitInc_Nm,VTQR_RrRateLimitDec_Nm,VTQR_ActREDUTrqUpLim_Nm,VTQR_ActREDUTrqLowLim_Nm
  Bus Selector1 : BusSelector  OutputSignals=task_time_s
  Constant : Constant  Value=ZERO_FLOAT
  Constant1 : Constant  Value=ZERO_FLOAT
  FirstOrderFilter : tqr/TQR/Determine Torque Request/TorqueArbitrament/TorqueSmooth/FirstOrderFilter
  FirstOrderFilter1 : tqr/TQR/Determine Torque Request/TorqueArbitrament/TorqueSmooth/FirstOrderFilter
  Limit : tqr/TQR/Determine Torque Request/TorqueArbitrament/TorqueSmooth/Limit
  Limit2 : tqr/TQR/Determine Torque Request/TorqueArbitrament/TorqueSmooth/Limit
  RateLimit : tqr/TQR/Determine Torque Request/TorqueArbitrament/TorqueSmooth/RateLimit
  RateLimit1 : tqr/TQR/Determine Torque Request/TorqueArbitrament/TorqueSmooth/RateLimit
  Unit Delay{1..4} (4 alike) : UnitDelay  SampleTime=-1
  VTQR_FrFirstOrderOutTqDelay_Nm : Outport
  VTQR_FEDUWhlTqReqSmoothDelay_Nm : Outport  Port=2
  VTQR_RampFEDUWhlTqReq_Nm : Outport  Port=3
  VTQR_RrFirstOrderOutTqDelay_Nm : Outport  Port=4
  VTQR_REDUWhlTqReqSmoothDelay_Nm : Outport  Port=5
  VTQR_RampREDUWhlTqReq_Nm : Outport  Port=6
  wires:
  [task_time_s] -> FirstOrderFilter/2
  Limit/1 -> [VTQR_RampFEDUWhlTqReq_Nm]  "VTQR_RampFEDUWhlTqReq_Nm"
  [VTQR_FrFirstOrderInpTs_c] -> FirstOrderFilter/3
  Constant/1 -> RateLimit/2
  Unit Delay3/1 -> [VTQR_FrFirstOrderOutTqDelay_Nm]  "VTQR_FrFirstOrderOutTqDelay_Nm"
  [VTQR_FrFirstOrderInpTq_Nm] -> FirstOrderFilter/1
  [VTQR_FrRateLimitDec_Nm] -> RateLimit/5
  RateLimit/1 -> Unit Delay1/1  "VTQR_FEDUWhlTqReqSmooth_Nm"
  FirstOrderFilter/1 -> Unit Delay3/1, RateLimit/1  "VTQR_FrFirstOrderOutTq_Nm"
  [VTQR_FrRateLimitInc_Nm] -> RateLimit/4
  Unit Delay1/1 -> [VTQR_FEDUWhlTqReqSmoothDelay_Nm], Limit/1  "VTQR_FEDUWhlTqReqSmoothDelay_Nm"
  [task_time_s] -> RateLimit/3
  [VTQR_RrFirstOrderInpTq_Nm] -> FirstOrderFilter1/1
  Unit Delay2/1 -> [VTQR_REDUWhlTqReqSmoothDelay_Nm], Limit2/1  "VTQR_REDUWhlTqReqSmoothDelay_Nm"
  [VTQR_RrRateLimitDec_Nm] -> RateLimit1/5
  [VTQR_RrRateLimitInc_Nm] -> RateLimit1/4
  [VTQR_ActREDUTrqLowLim_Nm] -> Limit2/3
  [VTQR_ActREDUTrqUpLim_Nm] -> Limit2/2
  [task_time_s] -> RateLimit1/3
  RateLimit1/1 -> Unit Delay2/1  "VTQR_REDUWhlTqReqSmooth_Nm"
  Limit2/1 -> [VTQR_RampREDUWhlTqReq_Nm]  "VTQR_RampREDUWhlTqReq_Nm"
  FirstOrderFilter1/1 -> Unit Delay4/1, RateLimit1/1  "VTQR_RrFirstOrderOutTq_Nm"
  [VTQR_RrFirstOrderInpTs_c] -> FirstOrderFilter1/3
  Constant1/1 -> RateLimit1/2
  Unit Delay4/1 -> [VTQR_RrFirstOrderOutTqDelay_Nm]  "VTQR_RrFirstOrderOutTqDelay_Nm"
  [task_time_s] -> FirstOrderFilter1/2
  VTQR_FrFirstOrderInpTq_Nm/1 -> [VTQR_FrFirstOrderInpTq_Nm]
  VTQR_RrFirstOrderInpTq_Nm/1 -> [VTQR_RrFirstOrderInpTq_Nm]
  BInpConvert_outputs/1 -> Bus Selector/1
  BSCPIn_outputs/1 -> Bus Selector1/1
  Bus Selector1/1 -> [task_time_s]  "<task_time_s>"
  Bus Selector/1 -> [VTQR_FrFirstOrderInpTs_c]  "<VTQR_FrFirstOrderInpTs_c>"
  Bus Selector/2 -> [VTQR_FrRateLimitInc_Nm]  "<VTQR_FrRateLimitInc_Nm>"
  Bus Selector/3 -> [VTQR_FrRateLimitDec_Nm]  "<VTQR_FrRateLimitDec_Nm>"
  Bus Selector/4 -> [VTQR_ActFEDUTrqUpLim_Nm]  "<VTQR_ActFEDUTrqUpLim_Nm>"
  Bus Selector/5 -> [VTQR_ActFEDUTrqLowLim_Nm]  "<VTQR_ActFEDUTrqLowLim_Nm>"
  Bus Selector/6 -> [VTQR_RrFirstOrderInpTs_c]  "<VTQR_RrFirstOrderInpTs_c>"
  Bus Selector/7 -> [VTQR_RrRateLimitInc_Nm]  "<VTQR_RrRateLimitInc_Nm>"
  Bus Selector/8 -> [VTQR_RrRateLimitDec_Nm]  "<VTQR_RrRateLimitDec_Nm>"
  Bus Selector/9 -> [VTQR_ActREDUTrqUpLim_Nm]  "<VTQR_ActREDUTrqUpLim_Nm>"
  Bus Selector/10 -> [VTQR_ActREDUTrqLowLim_Nm]  "<VTQR_ActREDUTrqLowLim_Nm>"
  [VTQR_FrFirstOrderOutTqDelay_Nm] -> VTQR_FrFirstOrderOutTqDelay_Nm/1
  [VTQR_FEDUWhlTqReqSmoothDelay_Nm] -> VTQR_FEDUWhlTqReqSmoothDelay_Nm/1
  [VTQR_RampFEDUWhlTqReq_Nm] -> VTQR_RampFEDUWhlTqReq_Nm/1
  [VTQR_RrFirstOrderOutTqDelay_Nm] -> VTQR_RrFirstOrderOutTqDelay_Nm/1
  [VTQR_REDUWhlTqReqSmoothDelay_Nm] -> VTQR_REDUWhlTqReqSmoothDelay_Nm/1
  [VTQR_RampREDUWhlTqReq_Nm] -> VTQR_RampREDUWhlTqReq_Nm/1
  [VTQR_ActFEDUTrqUpLim_Nm] -> Limit/2
  [VTQR_ActFEDUTrqLowLim_Nm] -> Limit/3
